simulink model "parte3_eje6_avr_sta1"  (R2017b)
settings: Solver=VariableStepAuto  StartTime=0.0  StopTime=50  RelTol=1e-3
values from neighbouring files (symbols this model uses):
  IFD = 0    [parte3_eje6_ESST1A.m]
  ILR = 2    [parte3_eje6_ESST1A.m]
  KA = 187    [parte3_DC1A_data.m]    (also in parte3_eje2_SMIB_Exc_graph.m = 1000; parte3_eje6_ESST1A.m = 51)
  KC = 0.2    [parte3_eje3_EXAC1.m]    (also in parte3_eje3_EXAC2.m; parte3_eje5_ESSTB.m = 0.1; parte3_eje6_ESST1A.m = 0.01)
  KF = 0.058    [parte3_DC1A_data.m]    (also in parte3_eje6_ESST1A.m = 0.1)
  KLR = 1    [parte3_eje6_ESST1A.m]
  TA = 0.89    [parte3_DC1A_data.m]    (also in parte3_eje2_SMIB_Exc_graph.m = 0.1; parte3_eje6_ESST1A.m = 0.01)
  TB = 0.06    [parte3_DC1A_data.m]    (also in parte3_eje6_ESST1A.m = 10)
  TB1 = 0.1    [parte3_eje6_ESST1A.m]
  TC = 0.173    [parte3_DC1A_data.m]    (also in parte3_eje6_ESST1A.m = 0.01)
  TC1 = 0.01    [parte3_eje6_ESST1A.m]
  TF = 0.62    [parte3_DC1A_data.m]    (also in parte3_eje6_ESST1A.m = 0.31)
  VIMAX = 0.2    [parte3_eje6_ESST1A.m]
  VIMIN = -0.2    [parte3_eje6_ESST1A.m]
  VRMAX = 1.7    [parte3_DC1A_data.m]    (also in parte3_eje5_ESSTB.m = 1; parte3_eje6_ESST1A.m = 3.4)
  VRMIN = -1.7    [parte3_DC1A_data.m]    (also in parte3_eje5_ESSTB.m = -0.87; parte3_eje6_ESST1A.m = -3.4)
  VT = 1    [parte3_eje6_ESST1A.m]
settings Model: Creator=cjuar  LastModifiedBy=cjuar

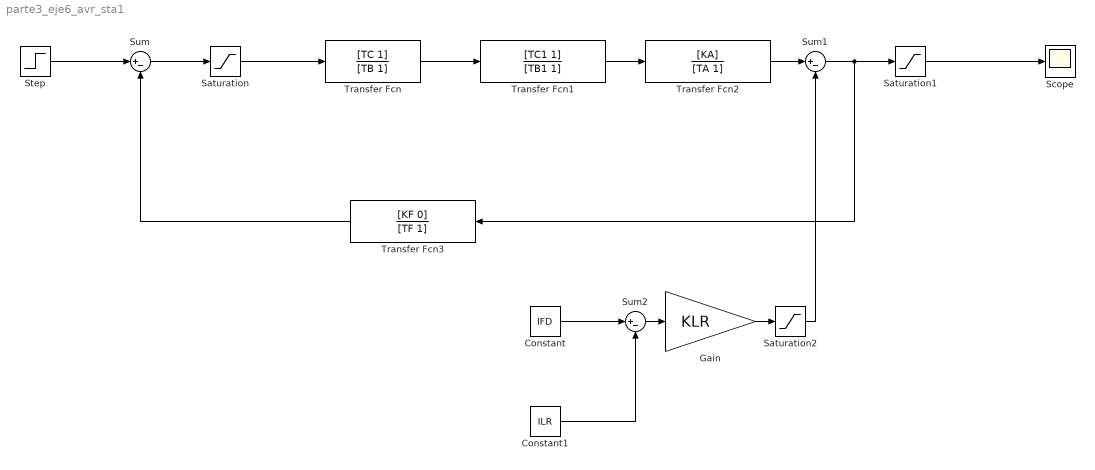
== system parte3_eje6_avr_sta1 ==
  Constant : Constant  Value=IFD
  Constant1 : Constant  Value=ILR
  Gain : Gain  Gain=KLR
  Saturation : Saturate  UpperLimit=VIMAX  LowerLimit=VIMIN
  Saturation1 : Saturate  UpperLimit=VT*VRMAX-KC*IFD  LowerLimit=VT*VRMIN
  Saturation2 : Saturate  UpperLimit=2000  LowerLimit=0
  Scope : Scope
  Step : Step  After=0.01  SampleTime=0
  Sum : Sum  Inputs=|+-
  Sum1 : Sum  Inputs=|+-
  Sum2 : Sum  Inputs=|+-
  Transfer Fcn : TransferFcn  Numerator=[TC 1]  Denominator=[TB 1]
  Transfer Fcn1 : TransferFcn  Numerator=[TC1 1]  Denominator=[TB1 1]
  Transfer Fcn2 : TransferFcn  Numerator=[KA]  Denominator=[TA 1]
  Transfer Fcn3 : TransferFcn  Numerator=[KF 0]  Denominator=[TF 1]
  wires:
  Step/1 -> Sum/1
  Sum/1 -> Saturation/1
  Saturation/1 -> Transfer Fcn/1
  Transfer Fcn/1 -> Transfer Fcn1/1
  Transfer Fcn2/1 -> Sum1/1
  Transfer Fcn3/1 -> Sum/2
  Sum2/1 -> Gain/1
  Constant/1 -> Sum2/1
  Constant1/1 -> Sum2/2
  Saturation1/1 -> Scope/1
  Sum1/1 -> Saturation1/1, Transfer Fcn3/1
  Transfer Fcn1/1 -> Transfer Fcn2/1
  Gain/1 -> Saturation2/1
  Saturation2/1 -> Sum1/2
